simulink model "mass_sim_HW_06"  (R2018a)
settings: Solver=ode45  StartTime=0.0  StopTime=50  MaxStep=1  RelTol=1e-3
InitFcn:
  | mass_spring_damper_param
undefined symbols (not defined in the file or in its folder): mass_spring_damper_animation, mass_spring_damper_ctrl, P
settings Model: Creator=canla  LastModifiedBy=canla
settings OptimizationCC: LifeSpan=inf

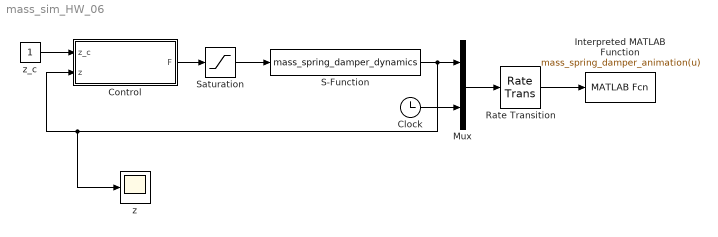
== system mass_sim_HW_06 ==
  Clock : Clock
  Control : Subsystem
  Interpreted MATLAB Function : MATLABFcn  MATLABFcn=mass_spring_damper_animation(u)  OutputDimensions=0
  Mux : Mux  Inputs=2
  Rate Transition : RateTransition  OutPortSampleTime=P.t_plot
  S-Function : S-Function  FunctionName=mass_spring_damper_dynamics  Parameters=P  SFunctionDeploymentMode=off  EnableBusSupport=off
  Saturation : Saturate  UpperLimit=P.F_max  LowerLimit=-P.F_max
  z : Scope
  z_c : Constant  SampleTime=P.Ts
  wires:
  z_c/1 -> Control/1(z_c)
  Rate Transition/1 -> Interpreted MATLAB Function/1
  Control/1(F) -> Saturation/1
  S-Function/1 -> z/1, Control/2(z), Mux/1
  Clock/1 -> Mux/2
  Mux/1 -> Rate Transition/1
  Saturation/1 -> S-Function/1

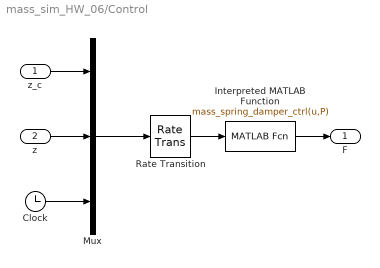
== system mass_sim_HW_06/Control ==
  z_c : Inport
  z : Inport  Port=2
  Clock : Clock
  Interpreted MATLAB Function : MATLABFcn  MATLABFcn=mass_spring_damper_ctrl(u,P)  OutputDimensions=1
  Mux : Mux  Inputs=3
  Rate Transition : RateTransition  OutPortSampleTime=P.Ts
  F : Outport
  wires:
  z_c/1 -> Mux/1
  z/1 -> Mux/2
  Clock/1 -> Mux/3
  Mux/1 -> Rate Transition/1
  Interpreted MATLAB Function/1 -> F/1
  Rate Transition/1 -> Interpreted MATLAB Function/1
